simulink model "kadai21"  (R2021b)
settings: Solver=VariableStepAuto  StartTime=0.0  StopTime=10.0  MaxStep=0.01  RelTol=1e-3
settings Model: Creator=is221042  LastModifiedBy=tomotomo

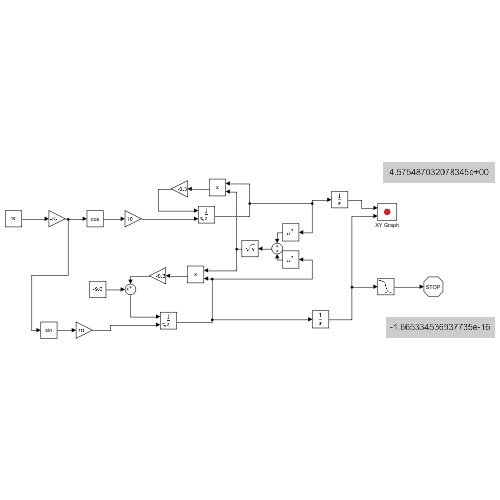
[thumbnail: Simulink's stored preview of the top-level diagram]
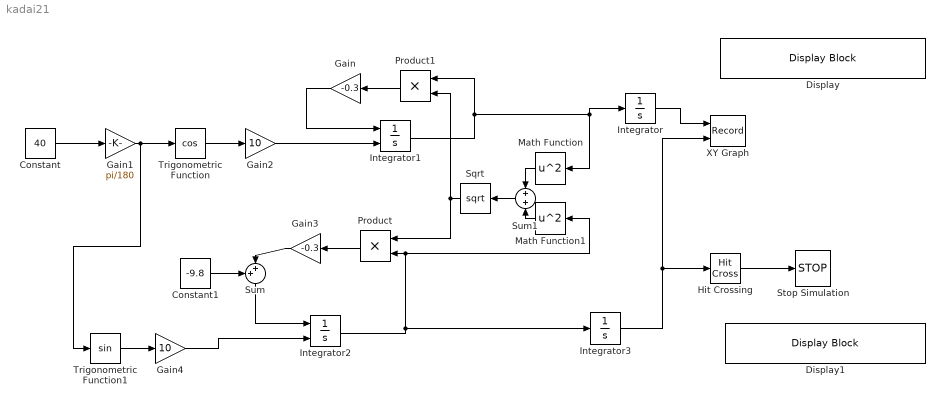
== system kadai21 ==
  Constant : Constant  Value=40
  Constant1 : Constant  Value=-9.8
  Display : DisplayBlock  LabelPosition=Hide  Format=longE  Transparency=1
  Display1 : DisplayBlock  LabelPosition=Hide  Format=longE  Transparency=1
  Gain : Gain  Gain=-0.3
  Gain1 : Gain  Gain=pi/180
  Gain2 : Gain  Gain=10
  Gain3 : Gain  Gain=-0.3
  Gain4 : Gain  Gain=10
  Hit Crossing : HitCross  HitCrossingDirection=falling
  Integrator : Integrator
  Integrator1 : Integrator  InitialConditionSource=external
  Integrator2 : Integrator  InitialConditionSource=external
  Integrator3 : Integrator
  Math Function : Math  Operator=square  SaturateOnIntegerOverflow=on
  Math Function1 : Math  Operator=square  SaturateOnIntegerOverflow=on
  Product : Product
  Product1 : Product
  Sqrt : Sqrt  SaturateOnIntegerOverflow=on
  Stop Simulation : Stop
  Sum : Sum  Inputs=++|
  Sum1 : Sum  Inputs=+|+
  Trigonometric Function : Trigonometry  Operator=cos
  Trigonometric Function1 : Trigonometry
  XY Graph : Record  FileSettingsInternal="{\"entries\":[{\"content\":{\"excelSettings\":{\"content\":{},\"type\":\"Streamout.ExcelSettings\"}},\"type\":\"Streamout.FileSettingStorage\",\"uuid\":\"5c2e8bae-098b-40b7-ab95-19e5ba179b7d\"}],\"packageUris\":[\"http://schema.mathworks.com/mf0/streamout_blocks/R2020a\"],\"version\":\"1.0\"}"  Layout=[1 1]  SignalsInternal="{\"entries\":[{\"content\":{\"signals\":[{\"content\":{\"blockPath\":[\"kadai21/XY Graph\"],\"channel\":[],\"dimensions\":[1],\"domain\":\"kadai21/XY Graph\",\"lineColor\":\"#a2142f\",\"plots\":[],\"port\":1,\"sid\":[\"\"],\"signalID\":588,\"signalName\":\"Integrator\"},\"type\":\"RecordBlkView.Signal\",\"uuid\":\"b6e63221-1431-4e42-9a7b-d8aed6d16f25\"},{\"content\":{\"blockPath\":[\"kadai21/XY Graph\"],\"channel\":[],\"dimensions\":[1],\"domain\":\"kadai21/XY Graph\",\"lineColor\":\"#139fff\",\"plots\":[],\"port\":2,\"sid\":[\"\"],\"signalID\":592,\"signalName\":\"Integrator3\"},\"type\":\"RecordBlkView.Signal\",\"uuid\":\"786dda1f-8314-4024-bb93-af73762a37e2\"}]},\"type\":\"RecordBlkView.InputSignals\",\"uuid\":\"b8ff8d21-0386-423d-a40b-e001c58a0463\"}],\"packageUris\":[\"http://schema.mathworks.com/mf0/streamout_blocks/R2020a\"],\"version\":\"1.0\"}"  VisualizationBindings="{\"xyplotplugin\":{\"info\":[{\"series\":[{\"bindingParametersList\":[{\"parameter\":\"X-Axis\",\"signalID\":588,\"signalName\":\"Integrator\"},{\"parameter\":\"Y-Axis\",\"signalID\":592,\"signalName\":\"Integrator3\"}],\"seriesID\":35719}],\"subplotID\":1}]}}"  CompatibilityTag=XY
  wires:
  Constant/1 -> Gain1/1
  Trigonometric Function/1 -> Gain2/1
  Gain1/1 -> Trigonometric Function1/1, Trigonometric Function/1
  Gain/1 -> Integrator1/1
  Gain2/1 -> Integrator1/2
  Constant1/1 -> Sum/1
  Gain3/1 -> Sum/2
  Trigonometric Function1/1 -> Gain4/1
  Sum/1 -> Integrator2/1
  Gain4/1 -> Integrator2/2
  Product/1 -> Gain3/1
  Product1/1 -> Gain/1
  Sqrt/1 -> Product/1, Product1/2
  Math Function/1 -> Sum1/1
  Math Function1/1 -> Sum1/2
  Sum1/1 -> Sqrt/1
  Integrator2/1 -> Math Function1/1, Product/2, Integrator3/1
  Integrator1/1 -> Integrator/1, Math Function/1, Product1/1
  Integrator/1 -> XY Graph/1
  Integrator3/1 -> XY Graph/2, Hit Crossing/1
  Hit Crossing/1 -> Stop Simulation/1
